simulink model "observations"  (R2021b)
settings: Solver=VariableStepAuto  StartTime=0.0  StopTime=10.0  RelTol=1e-3
settings Model: Creator=mluser  LastModifiedBy=mluser

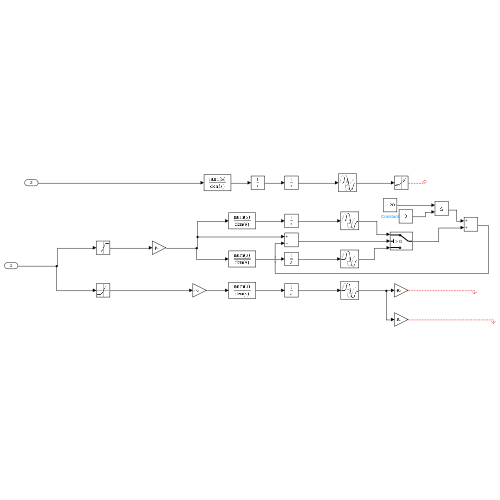
[thumbnail: Simulink's stored preview of the top-level diagram]
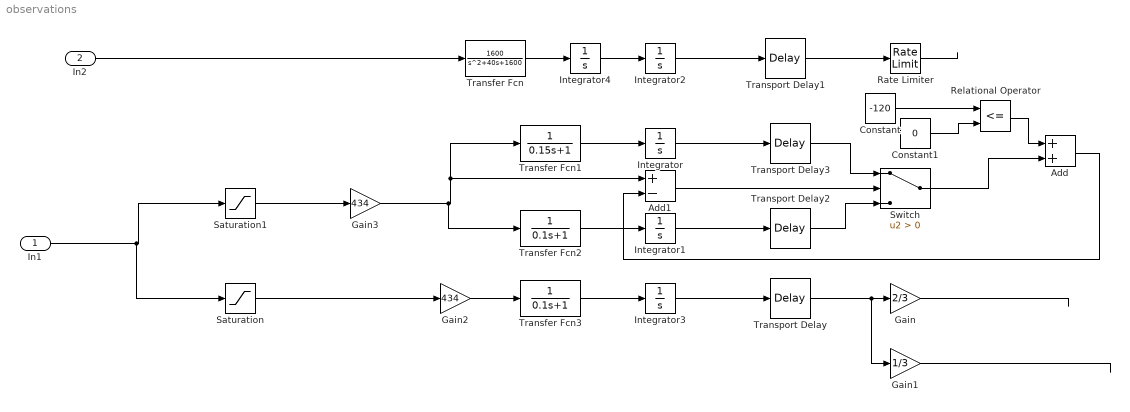
== system observations ==
  In1 : Inport
  In2 : Inport  Port=2
  Add : Sum
  Add1 : Sum  Inputs=+-
  Constant : Constant  Value=-120
  Constant1 : Constant  Value=0
  Gain : Gain  Gain=2/3
  Gain1 : Gain  Gain=1/3
  Gain2 : Gain  Gain=434
  Gain3 : Gain  Gain=434
  Integrator{,1..4} (5 alike) : Integrator
  Rate Limiter : RateLimiter  SampleTimeMode=inherited
  Relational Operator : RelationalOperator  Operator=<=  OutDataTypeStr=boolean  RndMeth=Simplest
  Saturation : Saturate  UpperLimit=0  LowerLimit=-20
  Saturation1 : Saturate  UpperLimit=20  LowerLimit=0
  Switch : Switch  Criteria=u2 > Threshold
  Transfer Fcn : TransferFcn  Numerator=[1600]  Denominator=[1 40 1600]
  Transfer Fcn1 : TransferFcn  Denominator=[0.15 1]
  Transfer Fcn2 : TransferFcn  Denominator=[0.1 1]
  Transfer Fcn3 : TransferFcn  Denominator=[0.1 1]
  Transport Delay : TransportDelay  DelayTime=0.1
  Transport Delay1 : TransportDelay  DelayTime=0.05
  Transport Delay2 : TransportDelay  DelayTime=0.1
  Transport Delay3 : TransportDelay  DelayTime=0.5
  wires:
  Transport Delay/1 -> Gain1/1, Gain/1
  Integrator3/1 -> Transport Delay/1
  Integrator1/1 -> Transport Delay2/1
  Integrator/1 -> Transport Delay3/1
  Integrator2/1 -> Transport Delay1/1
  Integrator4/1 -> Integrator2/1
  Transfer Fcn1/1 -> Integrator/1
  Transfer Fcn2/1 -> Integrator1/1
  Transfer Fcn3/1 -> Integrator3/1
  Transfer Fcn/1 -> Integrator4/1
  Transport Delay3/1 -> Switch/1
  Transport Delay2/1 -> Switch/3
  Saturation/1 -> Gain2/1
  Gain2/1 -> Transfer Fcn3/1
  Transport Delay1/1 -> Rate Limiter/1
  Rate Limiter/1 -> ?
  Gain/1 -> ?
  Gain1/1 -> ?
  In2/1 -> Transfer Fcn/1
  In1/1 -> Saturation/1, Saturation1/1
  Saturation1/1 -> Gain3/1
  Gain3/1 -> Transfer Fcn2/1, Add1/1, Transfer Fcn1/1
  Switch/1 -> Add/2
  Add/1 -> Add1/2
  Add1/1 -> Switch/2
  Constant/1 -> Relational Operator/1
  Constant1/1 -> Relational Operator/2
  Relational Operator/1 -> Add/1
